simulink model "ex7busLongLine_sim"  (R2014b)
settings: Solver=ode45  SolverMode=SingleTasking  StartTime=0.0  StopTime=5  MaxStep=0.0005  RelTol=1e-07
values from neighbouring files (symbols this model uses):
  bus1_vd = 2^0.5*1e3    (= 1414.21356237)    [ex3busPV.m]    (also in exLongLinePV.m = 141421.356237)
  C2 = 0.1*(len12/NN12+len23/NN23+len25/NN25)*Cx    (= 7.75146666667e-08)    [ex7busLongLine.m]
  C3 = 0.1*(len23/NN23+len34/NN34)*Cx    (= 3.50675e-08)    [ex7busLongLine.m]
  C4 = 0.1*(len14/NN14+len34/NN34+len46/NN46)*Cx    (= 9.28655e-08)    [ex7busLongLine.m]
  C5 = 0.1*(len25/NN25)*Cx    (= 2.39416666667e-08)    [ex7busLongLine.m]
  C6 = 0.1*(len46/NN46+len67/NN67)*Cx    (= 4.85875e-08)    [ex7busLongLine.m]
  C7 = 0.1*(len67/NN67)*Cx    (= 2.66175e-08)    [ex7busLongLine.m]
  CL2 = -CL2    [ex7busLongLine.m]
  CL3 = -CL3    [ex7busLongLine.m]
  CL6 = -CL6    [ex7busLongLine.m]
  CL7 = -CL7    [ex7busLongLine.m]
  DL2 = -DL2    [ex7busLongLine.m]
  DL3 = -DL3    [ex7busLongLine.m]
  DL6 = -DL6    [ex7busLongLine.m]
  DL7 = -DL7    [ex7busLongLine.m]
  droop_Pref = 0.25*Pbase    (= 75000000)    [ex7busLongLine.m]    (also in exDroopA.m = mpc.gen(2:end,PG)*1e6; exDroopB.m = mpc.gen(:,PG)*1e6; exSyncGenPVinv.m = droop_Pref( [1:(synrp-1),(synrp+1):end]  ))
  droop_R = DROOP_R_GAIN_CNST./Prt    [ex7busLongLine.m]    (also in exDroopA.m; exDroopB.m)
  Epv = 22e3    (= 22000)    [ex7busLongLine.m]
  If_dc = 0.2*Prt./Ert    [ex14busSGandPV.m]    (also in ex7busLongLine.m = Prt./(60*Vf_dc); exDroopA.m = Prt./(60*Vf_dc); exDroopB.m = Prt./(60*Vf_dc); exSyncGenPVinv.m)
  Jpv = JPV_CNST*Ppvrt/ws    (= 95.4929658551)    [ex7busLongLine.m]
  Kd = KD_GAIN_CNST*J*ws    [ex14busSGandPV.m]    (also in ex2busStability.m = 24000; ex7busLongLine.m; ex9busSG.m; exDroopA.m)
  Kdpv = KDPV_CNST*Jpv*ws    (= 6000000)    [ex7busLongLine.m]
  L0 = 0.1*Ld    [ex14busSGandPV.m]    (also in ex7busLongLine.m; exDroopA.m; exDroopB.m; exSyncGenPVinv.m)
  Laf = (2^0.5)*Ert./(ws*If_dc)    [ex14busSGandPV.m]    (also in ex7busLongLine.m; exDroopA.m; exDroopB.m; exSyncGenPVinv.m = (2^0.5)*5*Ert.^2./(ws*Prt))
  Lb2 = 2*Ld.*Lff - 3*Laf.^2    [ex14busSGandPV.m]    (also in ex7busLongLine.m; exDroopA.m; exDroopB.m; exSyncGenPVinv.m)
  Ld = 0.6*Lpu    [ex14busSGandPV.m]    (also in ex7busLongLine.m = 0.3*Lpu; exDroopA.m = 0.3*Lpu; exDroopB.m = 0.3*Lpu; exSyncGenPVinv.m)
  Lff = 2*Laf.^2./Ld    [ex14busSGandPV.m]    (also in ex7busLongLine.m; exDroopA.m; exDroopB.m; exSyncGenPVinv.m)
  Lq = Ld    [ex14busSGandPV.m]    (also in ex7busLongLine.m; exDroopA.m; exDroopB.m; exSyncGenPVinv.m)
  Lspv = 0.1*Epv^2/(Ppvrt*ws)    (= 0.00256769974855)    [ex7busLongLine.m]
  PG5 = 0.8*Ppvrt    (= 48000000)    [ex7busLongLine.m]
  poles_2Jws = poles./(2*J*ws)    [ex14busSGandPV.m]    (also in ex2busStability.m = poles./(2*ws*J); ex7busLongLine.m; ex9busSG.m = poles./(2*ws*J); exDroopA.m)
  Ra = 0.05*Ert.^2./Prt    [ex14busSGandPV.m]    (also in ex7busLongLine.m = 0.01*Ert.^2./Prt; exDroopA.m = 0.01*Ert.^2./Prt; exDroopB.m = 0.01*Ert.^2./Prt; exSyncGenPVinv.m)
  rel_step_4 = 0.5    [ex7busLongLine.m]
  rel_step_5 = -0.5    [ex7busLongLine.m]
  Rf = Lff/1.2    [ex14busSGandPV.m]    (also in ex7busLongLine.m = Vf_dc./If_dc; exDroopA.m = Vf_dc./If_dc; exDroopB.m = Vf_dc./If_dc; exSyncGenPVinv.m)
  tratio4 = 22e3 / Vbase    (= 0.136645962733)    [ex7busLongLine.m]
  tratio5 = 22e3 / Vbase    (= 0.136645962733)    [ex7busLongLine.m]
  tss2 = 4.5    [ex7busLongLine.m]
  tss3 = 1e9    (= 1000000000)    [ex7busLongLine.m]
  tss4 = 1e9    (= 1000000000)    [ex7busLongLine.m]
  tss5 = 4    [ex7busLongLine.m]
  tss6 = 1e9    (= 1000000000)    [ex7busLongLine.m]
  tss7 = 1e9    (= 1000000000)    [ex7busLongLine.m]
  Vbase = 161e3    (= 161000)    [ex7busLongLine.m]
  Vf_dc = If_dc.*Rf    [ex14busSGandPV.m]    (also in ex7busLongLine.m = 500 * ones(size(Ert)); exDroopA.m = 500 * ones(size(Ert)); exDroopB.m = 500 * ones(size(Ert)); exSyncGenPVinv.m)
  vinf_0 = 0    [ex14busSGandPV.m]    (also in ex7busLongLine.m; exDroopA.m; exSyncGenPVinv.m)
  vinf_d = (2^0.5)*mpcA.bus(1,VM)*baseV    [ex14busSGandPV.m]    (also in ex7busLongLine.m = 250457.221896; exDroopA.m = (2^0.5)*mpc.bus(1,VM)*baseV(1); exSyncGenPVinv.m = (2^0.5)*mpc.bus(1,VM)*baseV(1))
  vinf_q = 0    [ex14busSGandPV.m]    (also in ex7busLongLine.m; exDroopA.m; exSyncGenPVinv.m)
  ws = 2*pi*50    (= 314.159265359)    [ex14busSGandPV.m]    (also in ex2busStability.m; ex3busPV.m; ex7busLongLine.m; ex9busSG.m)
undefined symbols (not defined in the file or in its folder): AL2, AL3, AL6, AL7, At12, At14, At23, At25, At34, At46, At67, BL2, BL3, BL6, BL7, Bt12, Bt14, Bt23, Bt25, Bt34, Bt46, Bt67, Ct12, Ct14, Ct23, Ct25, Ct34, Ct46, Ct67, Dt12, Dt14, Dt23, Dt25, Dt34, Dt46, Dt67, full
(part 2 of 2)

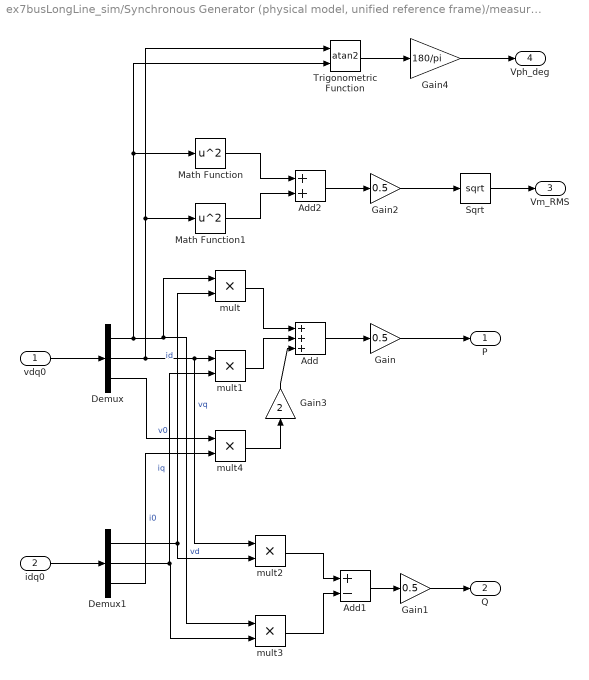
== system ex7busLongLine_sim/Synchronous Generator (physical model, unified reference frame)/measurements ==
  vdq0 : Inport
  idq0 : Inport  Port=2
  Add : Sum  Inputs=+++
  Add1 : Sum  Inputs=+-
  Add2 : Sum
  Demux : Demux  Outputs=3
  Demux1 : Demux  Outputs=3
  Gain : Gain  Gain=0.5
  Gain1 : Gain  Gain=0.5
  Gain2 : Gain  Gain=0.5
  Gain3 : Gain  Gain=2
  Gain4 : Gain  Gain=180/pi
  Math Function : Math  Operator=square  SaturateOnIntegerOverflow=on
  Math Function1 : Math  Operator=square  SaturateOnIntegerOverflow=on
  Sqrt : Sqrt  SaturateOnIntegerOverflow=on
  Trigonometric Function : Trigonometry  Operator=atan2
  mult{,1..4} (5 alike) : Product  Inputs=**
  P : Outport
  Q : Outport  Port=2
  Vm_RMS : Outport  Port=3
  Vph_deg : Outport  Port=4
  wires:
  idq0/1 -> Demux1/1
  vdq0/1 -> Demux/1
  Demux/1 -> Math Function/1, Trigonometric Function/2, mult3/1, mult/1  "vd"
  Demux/2 -> Trigonometric Function/1, Math Function1/1, mult2/1, mult1/1  "vq"
  Demux1/1 -> mult/2, mult2/2  "id"
  Demux1/2 -> mult3/2, mult1/2  "iq"
  Demux/3 -> mult4/1  "v0"
  Demux1/3 -> mult4/2  "i0"
  mult/1 -> Add/1
  mult1/1 -> Add/2
  Add/1 -> Gain/1
  mult2/1 -> Add1/1
  mult3/1 -> Add1/2
  Add1/1 -> Gain1/1
  Sqrt/1 -> Vm_RMS/1
  Math Function/1 -> Add2/1
  Math Function1/1 -> Add2/2
  Add2/1 -> Gain2/1
  Gain2/1 -> Sqrt/1
  Gain/1 -> P/1
  Gain1/1 -> Q/1
  mult4/1 -> Gain3/1
  Gain3/1 -> Add/3
  Trigonometric Function/1 -> Gain4/1
  Gain4/1 -> Vph_deg/1

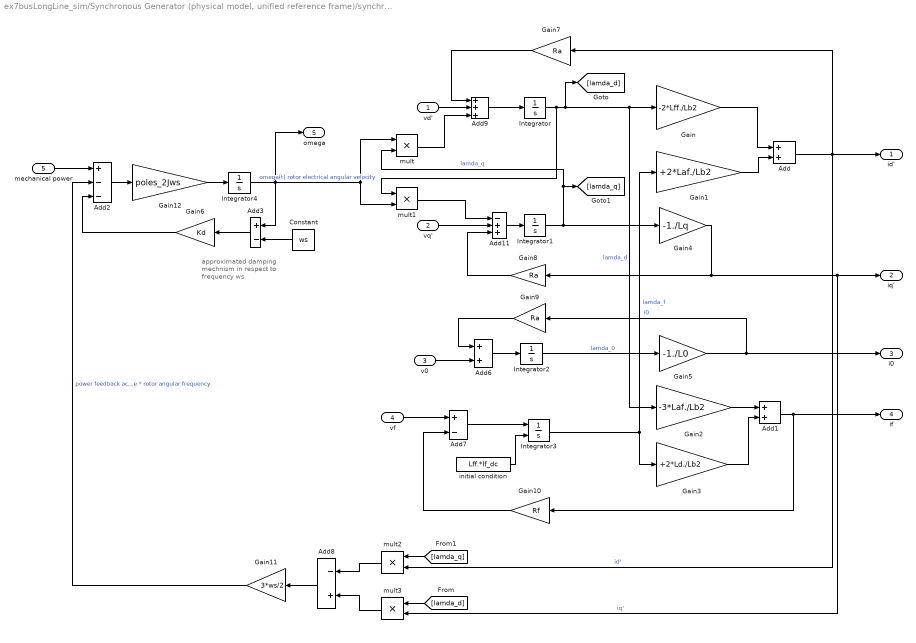
== system ex7busLongLine_sim/Synchronous Generator (physical model, unified reference frame)/synchronous machine dq0 model reference angle is teta(t) = rotor electrical angle ==
  note: approximated damping
      | mechnism in respect to
      | frequency ws
  vd' : Inport
  vq' : Inport  Port=2
  v0 : Inport  Port=3
  vf : Inport  Port=4
  mechanical power : Inport  Port=5
  Add : Sum
  Add1 : Sum
  Add11 : Sum  Inputs=-++
  Add2 : Sum  Inputs=+--
  Add3 : Sum  Inputs=+-
  Add6 : Sum
  Add7 : Sum  Inputs=+-
  Add8 : Sum  Inputs=-+
  Add9 : Sum  Inputs=+++
  Constant : Constant  Value=ws
  Gain : Gain  Gain=-2*Lff./Lb2
  Gain1 : Gain  Gain=+2*Laf./Lb2
  Gain10 : Gain  Gain=Rf
  Gain11 : Gain  Gain=3*ws/2
  Gain12 : Gain  Gain=poles_2Jws
  Gain2 : Gain  Gain=-3*Laf./Lb2
  Gain3 : Gain  Gain=+2*Ld./Lb2
  Gain4 : Gain  Gain=-1./Lq
  Gain5 : Gain  Gain=-1./L0
  Gain6 : Gain  Gain=Kd
  Gain7 : Gain  Gain=Ra
  Gain8 : Gain  Gain=Ra
  Gain9 : Gain  Gain=Ra
  Integrator : Integrator
  Integrator1 : Integrator
  Integrator2 : Integrator
  Integrator3 : Integrator  InitialConditionSource=external  InitialCondition=Lff(1)*If_dc(1)
  Integrator4 : Integrator  InitialCondition=ws
  initial condition : Constant  Value=Lff.*If_dc
  mult{,1..3} (4 alike) : Product  Inputs=**
  id' : Outport
  iq' : Outport  Port=2
  i0 : Outport  Port=3
  if : Outport  Port=4
  omega : Outport  Port=5
  wires:
  Gain1/1 -> Add/2
  Add6/1 -> Integrator2/1
  mechanical power/1 -> Add2/1
  Gain6/1 -> Add2/3
  Integrator/1 -> mult1/1, Gain2/1, Gain/1, [lamda_d]  "lamda_d"
  Gain5/1 -> i0/1, Gain9/1  "i0"
  Integrator1/1 -> Gain4/1, [lamda_q], mult/2  "lamda_q"
  Integrator2/1 -> Gain5/1  "lamda_0"
  Integrator3/1 -> Gain1/1, Gain3/1  "lamda_f"
  Add1/1 -> if/1, Gain10/1
  Gain4/1 -> iq'/1, mult3/2, Gain8/1  "iq'"
  Add/1 -> mult2/2, id'/1, Gain7/1  "id'"
  Gain/1 -> Add/1
  vf/1 -> Add7/1
  Add7/1 -> Integrator3/1
  Gain9/1 -> Add6/1
  Add8/1 -> Gain11/1
  Gain11/1 -> Add2/2  "power feedback acting to slow the rotor = Torque * rotor angular frequency"
  Gain8/1 -> Add11/3
  mult/1 -> Add9/3
  mult1/1 -> Add11/1
  Add9/1 -> Integrator/1
  vd'/1 -> Add9/2
  Gain3/1 -> Add1/2
  Gain2/1 -> Add1/1
  Gain10/1 -> Add7/2
  Add11/1 -> Integrator1/1
  Gain7/1 -> Add9/1
  mult3/1 -> Add8/2
  mult2/1 -> Add8/1
  v0/1 -> Add6/2
  Add3/1 -> Gain6/1
  Constant/1 -> Add3/2
  vq'/1 -> Add11/2
  [lamda_q] -> mult2/1
  [lamda_d] -> mult3/1
  Integrator4/1 -> omega/1, Add3/1, mult1/2, mult/1  "omega(t) rotor electrical angular velocity"
  Add2/1 -> Gain12/1
  Gain12/1 -> Integrator4/1
  initial condition/1 -> Integrator3/2

== system ex7busLongLine_sim/photovoltaic generator simple virtual inertia control based on dq0 quantities /series inductance + resistance ==
  vd1 : Inport
  vd2 : Inport  Port=2
  vq1 : Inport  Port=3
  vq2 : Inport  Port=4
  Add : Sum  Inputs=+-
  Add1 : Sum  Inputs=+-
  Add2 : Sum  Inputs=-++
  Add3 : Sum  Inputs=-+-
  Gain1 : Gain  Gain=1/Lspv
  Gain2 : Gain  Gain=1/Lspv
  Gain3 : Gain  Gain=ws
  Gain4 : Gain  Gain=ws
  Gain5 : Gain  Gain=Rspv/Lspv
  Gain7 : Gain  Gain=Rspv/Lspv
  Integrator : Integrator
  Integrator1 : Integrator
  id : Outport
  iq : Outport  Port=2
  wires:
  vd1/1 -> Add/1
  vd2/1 -> Add/2
  vq1/1 -> Add1/1
  vq2/1 -> Add1/2
  Add/1 -> Gain2/1
  Add1/1 -> Gain1/1
  Integrator/1 -> Gain4/1, id/1, Gain5/1
  Integrator1/1 -> Gain7/1, Gain3/1, iq/1
  Add2/1 -> Integrator/1
  Add3/1 -> Integrator1/1
  Gain3/1 -> Add2/3
  Gain2/1 -> Add2/2
  Gain4/1 -> Add3/1
  Gain1/1 -> Add3/2
  Gain5/1 -> Add2/1
  Gain7/1 -> Add3/3
